simulink model "sensorModel"  (R2025b)
settings: Solver=ode2  StartTime=0.0  StopTime=1  FixedStep=1/100  RelTol=1e-3  EnableMultiTasking=on
PreLoadFcn:
  | stepsize_sens = evalin('base', get_param(bdroot, 'FixedStep'));
undefined symbols (not defined in the file or in its folder): defaultConsts, DiscIntNeverNeededParam, sensors, vehicle
libraries: simulink x2, aerolibatmos2 x1
settings Model: Creator=ac112430  LastModifiedBy=ac124458
settings SolverCC: AlgebraicLoopSolver=TrustRegion
settings DataIOCC: ReturnWorkspaceOutputs=off
settings OptimizationCC: LifeSpan=inf
settings DebuggingCC: UnconnectedInputMsg=warning  UnconnectedOutputMsg=warning  UnconnectedLineMsg=warning  SFExecutionAtInitializationDiag=none  ArithmeticOperatorsInVariantConditions=warning
settings HardwareCC: ProdBitPerSizeT=32.0  ProdBitPerPtrDiffT=32.0  ProdWordSize=32.0  ProdHWDeviceType=Specified
settings ModelReferenceCC: EnableRefExpFcnMdlSchedulingChecks=on  ModelReferenceNumInstancesAllowed=Single
settings SFSimCC: SimUseLocalCustomCode=off  CustomCodeUndefinedFunction=UseInterfaceOnly
settings RTWCC: RTWUseLocalCustomCode=off  GPUComputeCapability=3.5
settings CodeAppCC: StateflowObjectComments=on
settings GRTTargetCC: SubcomponentCodeInterfacePackaging=Nonreusable function

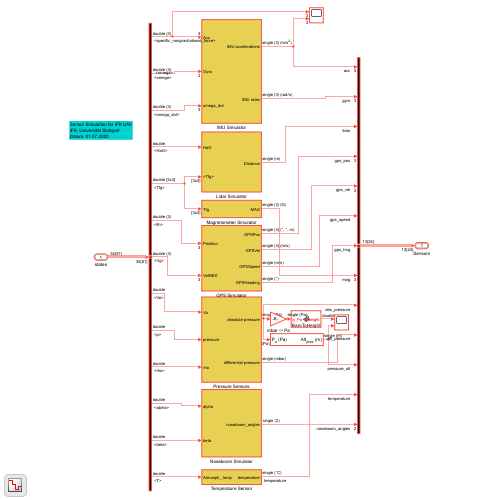
[thumbnail: Simulink's stored preview of the top-level diagram]
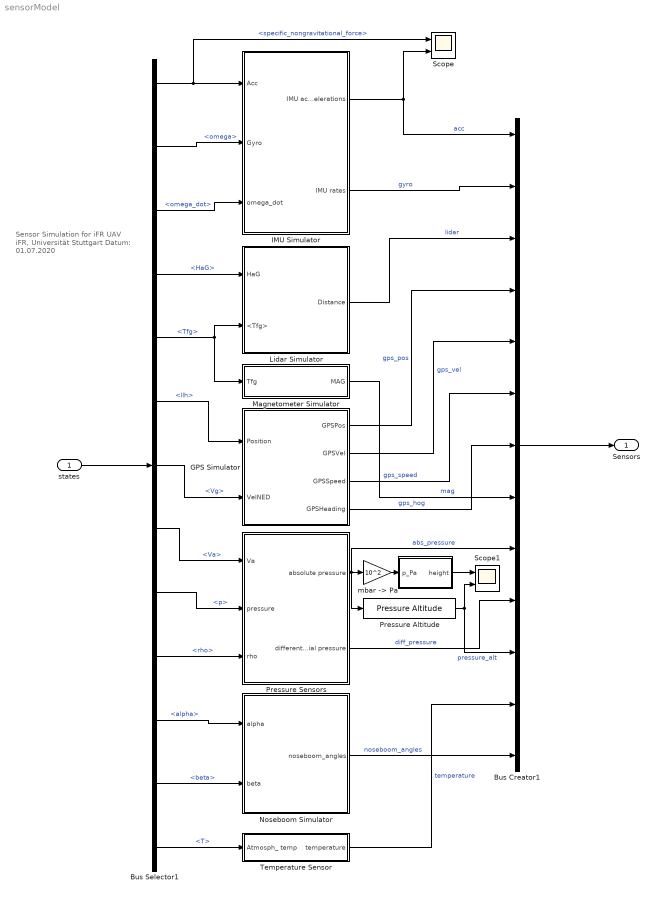
== system sensorModel ==
  note: Sensor Simulation for iFR UAV
      | iFR, Universität Stuttgart
      | Datum: 01.07.2020
  states : Inport  OutDataTypeStr=Bus: fmBus
  " " : MATLAB Function  TreatAsAtomicUnit=on
  Bus Creator1 : BusCreator  Inputs=13  OutDataTypeStr=Bus: sensorBus
      settings: InheritFromInputs=off
  Bus Selector1 : BusSelector  OutputSignals=utilityBus.specific_nongravitational_force,rigidbodyBus.omega,utilityBus.omega_dot,utilityBus.HaG,rigidbodyBus.Tfg,rigidbodyBus.llh,rigidbodyBus.Vg,atmosBus.Va,atmosBus.p,atmosBus.rho,atmosBus.alpha,atmosBus.beta,atmosBus.T
  GPS Simulator : Subsystem
  IMU Simulator : Subsystem
  Lidar Simulator : Subsystem
  Magnetometer Simulator : Subsystem
  Noseboom Simulator : Subsystem
  Pressure Altitude : aerolibatmos2/Pressure Altitude  units=Metric (MKS)  action=Warning
  Pressure Sensors : Subsystem
  Scope : Scope  NumInputPorts=2
      settings: ActiveDisplayYMinimum=-13.26607  ActiveDisplayYMaximum=18.32834
  Scope1 : Scope  NumInputPorts=2
      settings: DataLoggingVariableName=ScopeData2
  Temperature Sensor : Subsystem
  "mbar -> Pa" : Gain  Gain=10^2
  Sensors : Outport  OutDataTypeStr=Bus: sensorBus
  wires:
  Temperature Sensor/1(temperature) -> Bus Creator1/12  "temperature"
  Pressure Sensors/1(absolute pressure) -> Bus Creator1/9, Pressure Altitude/1, "mbar -> Pa"/1  "abs_pressure"
  GPS Simulator/2(GPSVel) -> Bus Creator1/5  "gps_vel"
  GPS Simulator/4(GPSHeading) -> Bus Creator1/7  "gps_hog"
  Magnetometer Simulator/1(MAG) -> Bus Creator1/8  "mag"
  Pressure Sensors/2(differential pressure) -> Bus Creator1/10  "diff_pressure"
  IMU Simulator/1(IMU accelerations) -> Bus Creator1/1, Scope/2  "acc"
  IMU Simulator/2(IMU rates) -> Bus Creator1/2  "gyro"
  Pressure Altitude/1 -> Bus Creator1/11, Scope1/2  "pressure_alt"
  Noseboom Simulator/1(noseboom_angles) -> Bus Creator1/13  "noseboom_angles"
  GPS Simulator/3(GPSSpeed) -> Bus Creator1/6  "gps_speed"
  GPS Simulator/1(GPSPos) -> Bus Creator1/4  "gps_pos"
  Bus Selector1/3 -> IMU Simulator/3(omega_dot)  "<omega_dot>"
  Bus Selector1/2 -> IMU Simulator/2(Gyro)  "<omega>"
  Bus Selector1/11 -> Noseboom Simulator/1(alpha)  "<alpha>"
  Bus Selector1/12 -> Noseboom Simulator/2(beta)  "<beta>"
  Bus Selector1/10 -> Pressure Sensors/3(rho)  "<rho>"
  states/1 -> Bus Selector1/1
  Bus Selector1/6 -> GPS Simulator/1(Position)  "<llh>"
  Bus Selector1/9 -> Pressure Sensors/2(pressure)  "<p>"
  Bus Selector1/5 -> Lidar Simulator/2(<Tfg>), Magnetometer Simulator/1(Tfg)  "<Tfg>"
  Bus Selector1/4 -> Lidar Simulator/1(HaG)  "<HaG>"
  Bus Selector1/8 -> Pressure Sensors/1(Va)  "<Va>"
  Bus Selector1/7 -> GPS Simulator/2(VelNED)  "<Vg>"
  Bus Selector1/1 -> Scope/1, IMU Simulator/1(Acc)  "<specific_nongravitational_force>"
  Bus Selector1/13 -> Temperature Sensor/1(Atmosph_ temp)  "<T>"
  Lidar Simulator/1(Distance) -> Bus Creator1/3  "lidar"
  "mbar -> Pa"/1 -> " "/1(p_Pa)
  " "/1(height) -> Scope1/1
  Bus Creator1/1 -> Sensors/1

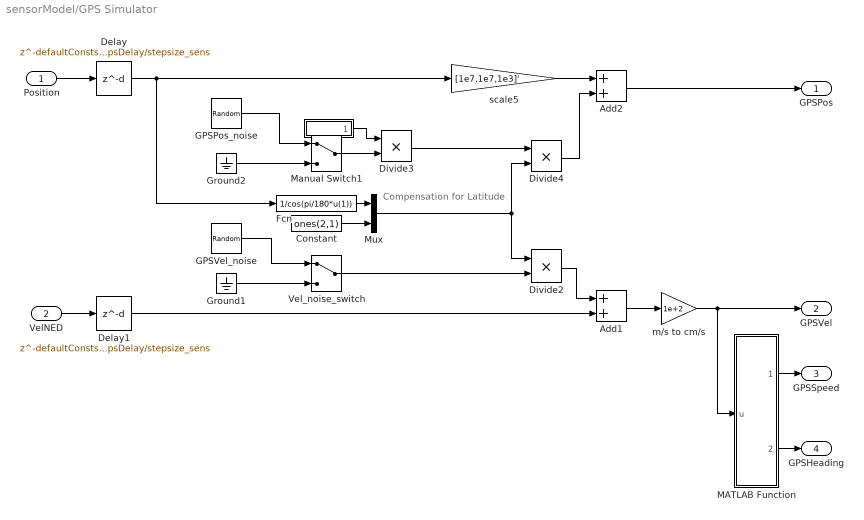
== system sensorModel/GPS Simulator ==
  note: Compensation for Latitude
  Position : Inport
  VelNED : Inport  Port=2
  "  " : MATLAB Function  TreatAsAtomicUnit=on
  Add1 : Sum
  Add2 : Sum  OutDataTypeStr=single
  Constant : Constant  Value=ones(2,1)
  Delay : Delay  DelayLength=defaultConsts.gpsDelay/stepsize_sens  InitialCondition=vehicle.pos0'*ones(1,defaultConsts.gpsDelay/stepsize_sens)
  Delay1 : Delay  DelayLength=defaultConsts.gpsDelay/stepsize_sens  InitialCondition=vehicle.pos0'*ones(1,defaultConsts.gpsDelay/stepsize_sens)
  Divide2 : Product  Inputs=**
  Divide3 : Product  Inputs=**
  Divide4 : Product  Inputs=**
  Fcn : Fcn  Expr=1/cos(pi/180*u(1))
  GPSPos_noise : RandomNumber  Variance=sensors.gps.sigmaPos.^2  Seed=[24522 237487 32748]
  GPSVel_noise : RandomNumber  Variance=sensors.gps.sigmaVel.^2  Seed=[127 2778 1883]
  Ground1 : Ground
  Ground2 : Ground
  MATLAB Function : MATLAB Function  TreatAsAtomicUnit=on
  Manual Switch1 : ManualSwitch
  Mux : Mux  Inputs=2
  Vel_noise_switch : ManualSwitch
  m/s to cm/s : Gain  Gain=1e+2  OutDataTypeStr=single
  scale5 : Gain  Gain=[1e7,1e7,1e3]'
  GPSPos : Outport  OutDataTypeStr=single  VectorParamsAs1DForOutWhenUnconnected=off
  GPSVel : Outport  Port=2  OutDataTypeStr=single  VectorParamsAs1DForOutWhenUnconnected=off
  GPSSpeed : Outport  Port=3  OutDataTypeStr=single  VectorParamsAs1DForOutWhenUnconnected=off
  GPSHeading : Outport  Port=4  OutDataTypeStr=single  VectorParamsAs1DForOutWhenUnconnected=off
  wires:
  Vel_noise_switch/1 -> Divide2/2
  Add1/1 -> m/s to cm/s/1
  VelNED/1 -> Delay1/1
  GPSVel_noise/1 -> Vel_noise_switch/1
  Ground1/1 -> Vel_noise_switch/2
  Delay1/1 -> Add1/2
  Manual Switch1/1 -> Divide3/2
  Delay/1 -> scale5/1, Fcn/1
  Position/1 -> Delay/1
  Ground2/1 -> Manual Switch1/2
  Mux/1 -> Divide2/1, Divide4/2
  Add2/1 -> GPSPos/1
  m/s to cm/s/1 -> GPSVel/1, MATLAB Function/1(u)
  MATLAB Function/1(speed) -> GPSSpeed/1
  MATLAB Function/2(heading) -> GPSHeading/1
  Divide2/1 -> Add1/1
  Divide3/1 -> Divide4/1
  GPSPos_noise/1 -> Manual Switch1/1
  Divide4/1 -> Add2/2
  Fcn/1 -> Mux/1
  Constant/1 -> Mux/2
  scale5/1 -> Add2/1
  "  "/1(ned2lla) -> Divide3/1

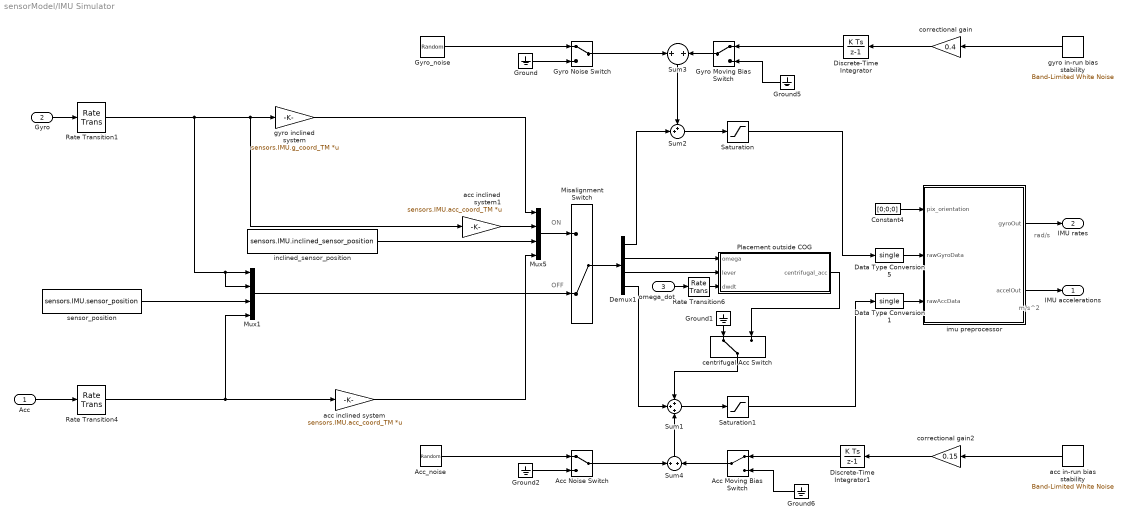
== system sensorModel/IMU Simulator ==
  note: ON
  note: OFF
  note: rad/s
  note: m/s^2
  Acc : Inport
  Gyro : Inport  Port=2
  omega_dot : Inport  Port=3
  Acc Moving Bias Switch : ManualSwitch
  Acc Noise Switch : ManualSwitch
  Acc_noise : RandomNumber  Mean=sensors.IMU.acc_initial_bias  Variance=sensors.IMU.acc_noise^2*[1 1 1]  Seed=[6 7 8]  SampleTime=sensors.IMU.timestep
  Constant4 : Constant  Value=[0;0;0]  OutDataTypeStr=single
  Data Type Conversion1 : DataTypeConversion  OutDataTypeStr=single  SaturateOnIntegerOverflow=off  RndMeth=Floor
  Data Type Conversion5 : DataTypeConversion  OutDataTypeStr=single  SaturateOnIntegerOverflow=off  RndMeth=Floor
  Demux1 : Demux
  Discrete-Time Integrator : DiscreteIntegrator  SampleTime=-1  ICPrevOutput=DiscIntNeverNeededParam  ICPrevScaledInput=DiscIntNeverNeededParam
  Discrete-Time Integrator1 : DiscreteIntegrator  SampleTime=-1  ICPrevOutput=DiscIntNeverNeededParam  ICPrevScaledInput=DiscIntNeverNeededParam
  Ground{,1..2,5..6} (5 alike) : Ground
  Gyro Moving Bias Switch : ManualSwitch
  Gyro Noise Switch : ManualSwitch
  Gyro_noise : RandomNumber  Mean=sensors.IMU.g_initial_bias  Variance=sensors.IMU.g_noise^2*[1 1 1]  Seed=[0 1 2]  SampleTime=sensors.IMU.timestep
  Misalignment Switch : ManualSwitch  CurrentSetting=0
  Mux1 : Mux
  Mux5 : Mux
  Placement outside COG : MATLAB Function  TreatAsAtomicUnit=on
  Rate Transition1 : RateTransition  OutPortSampleTime=sensors.IMU.timestep
  Rate Transition4 : RateTransition  OutPortSampleTime=sensors.IMU.timestep
  Rate Transition6 : RateTransition  OutPortSampleTime=stepsize_sens
  Saturation : Saturate  UpperLimit=sensors.IMU.g_range  LowerLimit=-sensors.IMU.g_range
  Saturation1 : Saturate  UpperLimit=sensors.IMU.acc_range  LowerLimit=-sensors.IMU.acc_range
  Sum1 : Sum  Inputs=+++
  Sum2 : Sum  Inputs=++|
  Sum3 : Sum
  Sum4 : Sum
  acc in-run bias stability : simulink/Sources/Band-Limited White Noise  Cov=sensors.IMU.acc_inrun_bias^2*[1 1 1]  Ts=sensors.IMU.timestep  seed=[40 31 56]
  acc inclined system : Gain  Gain=sensors.IMU.acc_coord_TM  Multiplication=Matrix(K*u)
  acc inclined system1 : Gain  Gain=sensors.IMU.acc_coord_TM  Multiplication=Matrix(K*u)
  centrifugal Acc Switch : ManualSwitch
  correctional gain : Gain  Gain=0.4
  correctional gain2 : Gain  Gain=0.15
  gyro in-run bias stability : simulink/Sources/Band-Limited White Noise  Cov=sensors.IMU.g_inrun_bias^2*[1 1 1]  Ts=sensors.IMU.timestep  seed=[21 30 27]
  gyro inclined system : Gain  Gain=sensors.IMU.g_coord_TM  Multiplication=Matrix(K*u)
  imu preprocessor : MATLAB Function  TreatAsAtomicUnit=on
  inclined_sensor_position : Constant  Value=sensors.IMU.inclined_sensor_position
  sensor_position : Constant  Value=sensors.IMU.sensor_position
  IMU accelerations : Outport  VectorParamsAs1DForOutWhenUnconnected=off
  IMU rates : Outport  Port=2  VectorParamsAs1DForOutWhenUnconnected=off
  wires:
  Sum2/1 -> Saturation/1
  Sum1/1 -> Saturation1/1
  Ground/1 -> Gyro Noise Switch/2
  Ground2/1 -> Acc Noise Switch/2
  Acc/1 -> Rate Transition4/1
  Rate Transition4/1 -> Mux1/4, acc inclined system/1
  centrifugal Acc Switch/1 -> Sum1/1
  Gyro/1 -> Rate Transition1/1
  Demux1/1 -> Sum2/2
  Ground1/1 -> centrifugal Acc Switch/1
  acc inclined system1/1 -> Mux5/2
  Misalignment Switch/1 -> Demux1/1
  acc inclined system/1 -> Mux5/4
  Mux1/1 -> Misalignment Switch/2
  Mux5/1 -> Misalignment Switch/1
  gyro inclined system/1 -> Mux5/1
  Demux1/4 -> Sum1/2
  Demux1/3 -> Placement outside COG/2(lever)
  inclined_sensor_position/1 -> Mux5/3
  Rate Transition1/1 -> gyro inclined system/1, acc inclined system1/1, Mux1/1, Mux1/2
  Gyro Noise Switch/1 -> Sum3/1
  Sum3/1 -> Sum2/1
  Acc Noise Switch/1 -> Sum4/1
  Sum4/1 -> Sum1/3
  Saturation/1 -> Data Type Conversion5/1
  Ground6/1 -> Acc Moving Bias Switch/2
  Discrete-Time Integrator1/1 -> Acc Moving Bias Switch/1
  Discrete-Time Integrator/1 -> Gyro Moving Bias Switch/1
  Ground5/1 -> Gyro Moving Bias Switch/2
  correctional gain/1 -> Discrete-Time Integrator/1
  Acc_noise/1 -> Acc Noise Switch/1
  Gyro_noise/1 -> Gyro Noise Switch/1
  gyro in-run bias stability/1 -> correctional gain/1
  acc in-run bias stability/1 -> correctional gain2/1
  Saturation1/1 -> Data Type Conversion1/1
  sensor_position/1 -> Mux1/3
  Demux1/2 -> Placement outside COG/1(omega)
  Placement outside COG/1(centrifugal_acc) -> centrifugal Acc Switch/2
  correctional gain2/1 -> Discrete-Time Integrator1/1
  Gyro Moving Bias Switch/1 -> Sum3/2
  Acc Moving Bias Switch/1 -> Sum4/2
  omega_dot/1 -> Rate Transition6/1
  Rate Transition6/1 -> Placement outside COG/3(dwdt)
  Data Type Conversion5/1 -> imu preprocessor/2(rawGyroData)
  Data Type Conversion1/1 -> imu preprocessor/3(rawAccData)
  Constant4/1 -> imu preprocessor/1(pix_orientation)
  imu preprocessor/1(gyroOut) -> IMU rates/1
  imu preprocessor/2(accelOut) -> IMU accelerations/1

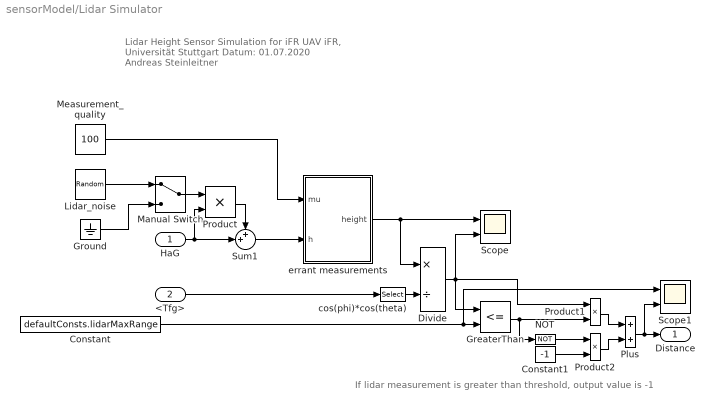
== system sensorModel/Lidar Simulator ==
  note: If lidar measurement is greater than threshold, output value is -1
  note: Lidar Height Sensor Simulation for iFR UAV
      | iFR, Universität Stuttgart
      | Datum: 01.07.2020
      |
      | Andreas Steinleitner
  HaG : Inport
  <Tfg> : Inport  Port=2
  Constant : Constant  Value=defaultConsts.lidarMaxRange
  Constant1 : Constant  Value=-1
  Divide : Product  Inputs=*/
  GreaterThan : RelationalOperator  Operator=<=  OutDataTypeStr=boolean  RndMeth=Simplest  InputSameDT=off
  Ground : Ground
  Lidar_noise : RandomNumber  Variance=sensors.lidar.sigma^2  Seed=29741  SampleTime=stepsize_sens
  Manual Switch : ManualSwitch
  Measurement_quality : Constant  Value=100
  NOT : Logic  Operator=NOT  AllPortsSameDT=off  OutDataTypeStr=boolean
  Plus : Sum  OutDataTypeStr=single
  Product : Product
  Product1 : Product
  Product2 : Product
  Scope : Scope  NumInputPorts=2
      settings: ActiveDisplayYMinimum=-38.99101  ActiveDisplayYMaximum=350.9191
  Scope1 : Scope  NumInputPorts=2
      settings: DataLoggingVariableName=ScopeData3
  Sum1 : Sum  Inputs=++|
  cos(phi)*cos(theta) : Selector  NumberOfDimensions=2  InputPortWidth=3  IndexOptions=Index vector (dialog),Index vector (dialog)  Indices=3,3  OutputSizes=1,1
  errant measurements : MATLAB Function  TreatAsAtomicUnit=on
  Distance : Outport  VectorParamsAs1DForOutWhenUnconnected=off
  wires:
  HaG/1 -> Product/2, Sum1/2
  Ground/1 -> Manual Switch/2
  Lidar_noise/1 -> Manual Switch/1
  Manual Switch/1 -> Product/1
  Product/1 -> Sum1/1
  <Tfg>/1 -> cos(phi)*cos(theta)/1
  cos(phi)*cos(theta)/1 -> Divide/2
  Measurement_quality/1 -> errant measurements/1(mu)
  Sum1/1 -> errant measurements/2(h)
  errant measurements/1(height) -> Scope/1, Divide/1
  Divide/1 -> Scope/2, GreaterThan/1, Product1/1
  Constant/1 -> Scope1/1, GreaterThan/2
  GreaterThan/1 -> NOT/1, Product1/2
  NOT/1 -> Product2/1
  Constant1/1 -> Product2/2
  Product1/1 -> Plus/1
  Product2/1 -> Plus/2
  Plus/1 -> Scope1/2, Distance/1

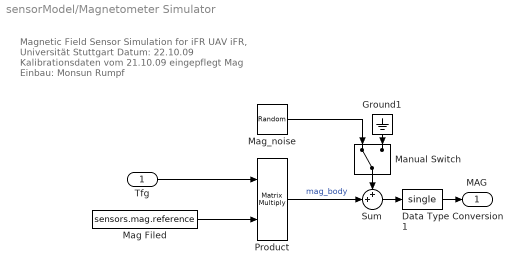
== system sensorModel/Magnetometer Simulator ==
  note: Magnetic Field Sensor Simulation for iFR UAV
      | iFR, Universität Stuttgart
      | Datum: 22.10.09
      |
      | Kalibrationsdaten vom 21.10.09 eingepflegt
      | Mag Einbau: Monsun Rumpf
  Tfg : Inport
  Data Type Conversion1 : DataTypeConversion  OutDataTypeStr=single  SaturateOnIntegerOverflow=off  RndMeth=Floor
  Ground1 : Ground
  Mag Filed : Constant  Value=sensors.mag.reference
  Mag_noise : RandomNumber  Variance=sensors.mag.sigma^2  Seed=[78234 3274 28736]  SampleTime=stepsize_sens
  Manual Switch : ManualSwitch
  Product : Product  Multiplication=Matrix(*)
  Sum : Sum  Inputs=++|
  MAG : Outport  VectorParamsAs1DForOutWhenUnconnected=off
  wires:
  Tfg/1 -> Product/1
  Product/1 -> Sum/2  "mag_body"
  Mag Filed/1 -> Product/2
  Sum/1 -> Data Type Conversion1/1
  Ground1/1 -> Manual Switch/2
  Mag_noise/1 -> Manual Switch/1
  Manual Switch/1 -> Sum/1
  Data Type Conversion1/1 -> MAG/1

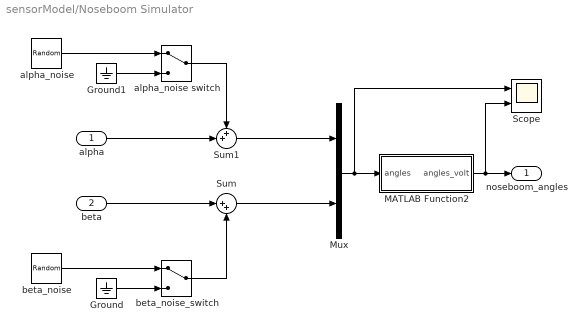
== system sensorModel/Noseboom Simulator ==
  alpha : Inport
  beta : Inport  Port=2
  Ground : Ground
  Ground1 : Ground
  MATLAB Function2 : MATLAB Function  TreatAsAtomicUnit=on
  Mux : Mux  Inputs=2
  Scope : Scope  NumInputPorts=2
      settings: ActiveDisplayYMinimum=-1.15354  ActiveDisplayYMaximum=0.87545
  Sum : Sum  Inputs=|++
  Sum1 : Sum  Inputs=++|
  alpha_noise : RandomNumber  Variance=deg2rad(0.5)^2  SampleTime=stepsize_sens
  alpha_noise switch : ManualSwitch
  beta_noise : RandomNumber  Variance=deg2rad(0.5)^2  SampleTime=stepsize_sens
  beta_noise_switch : ManualSwitch
  noseboom_angles : Outport  VectorParamsAs1DForOutWhenUnconnected=off
  wires:
  alpha/1 -> Sum1/2
  Sum1/1 -> Mux/1
  beta/1 -> Sum/1
  alpha_noise switch/1 -> Sum1/1
  beta_noise_switch/1 -> Sum/2
  Sum/1 -> Mux/2
  alpha_noise/1 -> alpha_noise switch/1
  beta_noise/1 -> beta_noise_switch/1
  Ground1/1 -> alpha_noise switch/2
  Ground/1 -> beta_noise_switch/2
  Mux/1 -> Scope/1, MATLAB Function2/1(angles)
  MATLAB Function2/1(angles_volt) -> Scope/2, noseboom_angles/1

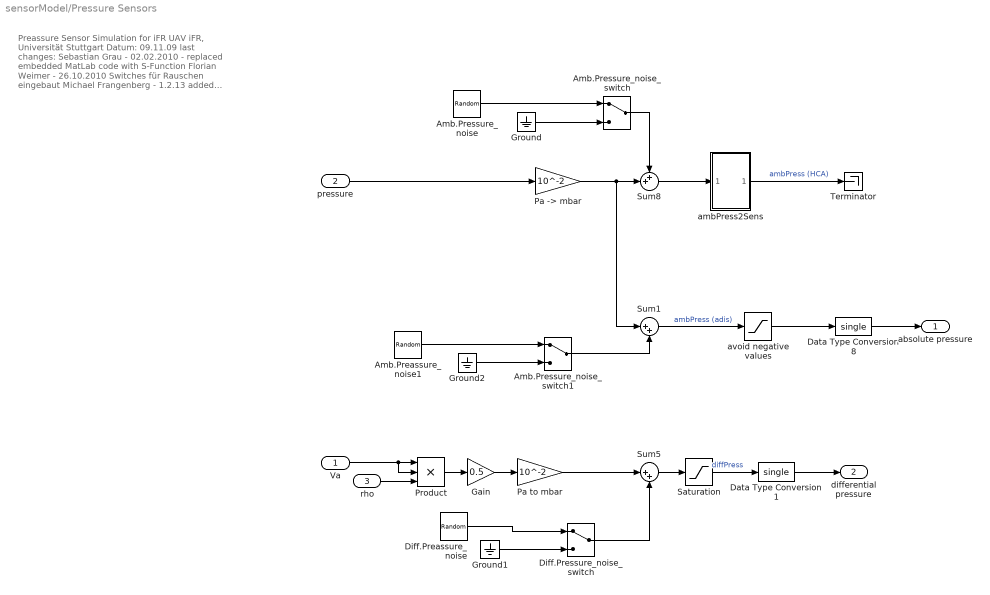
== system sensorModel/Pressure Sensors ==
  note: Preassure Sensor Simulation for iFR UAV
      | iFR, Universität Stuttgart
      | Datum: 09.11.09
      |
      | last changes:
      | Sebastian Grau - 02.02.2010 - replaced
      | embedded MatLab code with S-Function
      | Florian Weimer - 26.10.2010 Switches für
      | Rauschen eingebaut
      | Michael Frangenberg - 1.2.13 added ADIS baro
      |
      | Comments:
      | - add random walk process to sensors
  Va : Inport
  pressure : Inport  Port=2
  rho : Inport  Port=3
  Amb.Preassure_noise1 : RandomNumber  Variance=sensors.airData.sigmaAdis^2  Seed=6234  SampleTime=stepsize_sens
  Amb.Pressure_noise : RandomNumber  Variance=sensors.airData.sigmaHCA^2  Seed=29741  SampleTime=stepsize_sens
  Amb.Pressure_noise_switch : ManualSwitch
  Amb.Pressure_noise_switch1 : ManualSwitch
  Data Type Conversion1 : DataTypeConversion  OutDataTypeStr=single  SaturateOnIntegerOverflow=off  RndMeth=Floor
  Data Type Conversion8 : DataTypeConversion  OutDataTypeStr=single  SaturateOnIntegerOverflow=off  RndMeth=Floor
  Diff.Preassure_noise : RandomNumber  Variance=sensors.airData.sigmaDiff^2  Seed=237  SampleTime=stepsize_sens
  Diff.Pressure_noise_switch : ManualSwitch
  Gain : Gain  Gain=0.5
  Ground : Ground
  Ground1 : Ground
  Ground2 : Ground
  "Pa -> mbar" : Gain  Gain=10^-2
  Pa to mbar : Gain  Gain=10^-2
  Product : Product  Inputs=3
  Saturation : Saturate  UpperLimit=inf  LowerLimit=0.05
  Sum1 : Sum  Inputs=|++
  Sum5 : Sum  Inputs=|++
  Sum8 : Sum  Inputs=++|
  Terminator : Terminator
  ambPress2Sens : Subsystem
  avoid negative values : Saturate  UpperLimit=100000000000  LowerLimit=0.1
  absolute pressure : Outport  VectorParamsAs1DForOutWhenUnconnected=off
  differential pressure : Outport  Port=2  VectorParamsAs1DForOutWhenUnconnected=off
  wires:
  Diff.Pressure_noise_switch/1 -> Sum5/2
  Amb.Pressure_noise_switch/1 -> Sum8/1
  Sum8/1 -> ambPress2Sens/1(In1)
  Sum5/1 -> Saturation/1
  ambPress2Sens/1(Out1) -> Terminator/1  "ambPress (HCA)"
  Saturation/1 -> Data Type Conversion1/1  "diffPress"
  Amb.Pressure_noise/1 -> Amb.Pressure_noise_switch/1
  Ground/1 -> Amb.Pressure_noise_switch/2
  Diff.Preassure_noise/1 -> Diff.Pressure_noise_switch/1
  Ground1/1 -> Diff.Pressure_noise_switch/2
  Amb.Pressure_noise_switch1/1 -> Sum1/2
  Amb.Preassure_noise1/1 -> Amb.Pressure_noise_switch1/1
  Ground2/1 -> Amb.Pressure_noise_switch1/2
  Sum1/1 -> avoid negative values/1  "ambPress (adis)"
  pressure/1 -> "Pa -> mbar"/1
  Va/1 -> Product/2, Product/1
  rho/1 -> Product/3
  Product/1 -> Gain/1
  Gain/1 -> Pa to mbar/1
  Pa to mbar/1 -> Sum5/1
  "Pa -> mbar"/1 -> Sum1/1, Sum8/2
  Data Type Conversion8/1 -> absolute pressure/1
  Data Type Conversion1/1 -> differential pressure/1
  avoid negative values/1 -> Data Type Conversion8/1

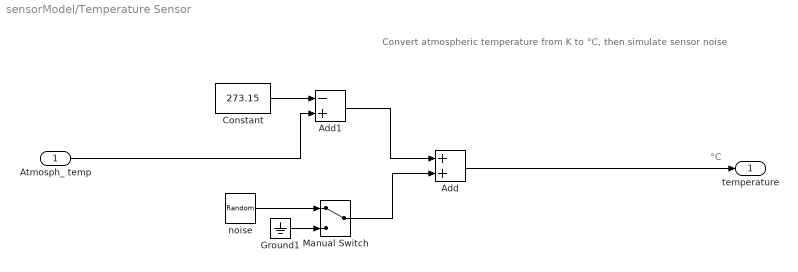
== system sensorModel/Temperature Sensor ==
  note: °C
  note: Convert atmospheric temperature from K to °C, then simulate sensor noise
  Atmosph_ temp : Inport
  Add : Sum  OutDataTypeStr=single
  Add1 : Sum  Inputs=-+  OutDataTypeStr=double
  Constant : Constant  Value=273.15
  Ground1 : Ground
  Manual Switch : ManualSwitch
  noise : RandomNumber  Variance=0.1^2  SampleTime=0.01
  temperature : Outport  OutDataTypeStr=single  VectorParamsAs1DForOutWhenUnconnected=off
  wires:
  Add/1 -> temperature/1
  Constant/1 -> Add1/1
  Atmosph_ temp/1 -> Add1/2
  Add1/1 -> Add/1
  Manual Switch/1 -> Add/2
  Ground1/1 -> Manual Switch/2
  noise/1 -> Manual Switch/1

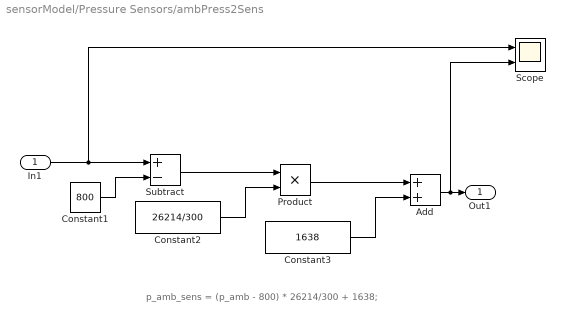
== system sensorModel/Pressure Sensors/ambPress2Sens ==
  note: p_amb_sens = (p_amb - 800) * 26214/300 + 1638;
  In1 : Inport
  Add : Sum
  Constant1 : Constant  Value=800
  Constant2 : Constant  Value=26214/300
  Constant3 : Constant  Value=1638
  Product : Product  RndMeth=Zero
  Scope : Scope  NumInputPorts=2
      settings: ActiveDisplayYMinimum=944.51744  ActiveDisplayYMaximum=961.03031
  Subtract : Sum  Inputs=+-
  Out1 : Outport  VectorParamsAs1DForOutWhenUnconnected=off
  wires:
  Subtract/1 -> Product/1
  Product/1 -> Add/1
  Constant3/1 -> Add/2
  Constant2/1 -> Product/2
  Constant1/1 -> Subtract/2
  In1/1 -> Scope/1, Subtract/1
  Add/1 -> Scope/2, Out1/1

== matlab function sensorModel/IMU Simulator/Placement outside COG ==
  data: omega input; centrifugal_acc output; lever input; dwdt input
function centrifugal_acc = fcn(omega, lever, dwdt)

%centrifugal acceleration is -omega x(omega x lever)
centrifugal_acc = zeros(3,1);
centrifugal_acc = cross(omega,cross(omega,lever)) + cross(dwdt, lever);

== matlab function sensorModel/GPS Simulator/MATLAB Function ==
  data: u input; speed output single; heading output single
function [speed,heading] = fcn(u)

speed = norm(u);
heading = atan2(u(2),u(1));

== matlab function sensorModel/Lidar Simulator/errant measurements ==
  data: mu input; h input; height output; sensors parameter
function height = fcn(mu,h,sensors)

maxHeight = 50;
height = h;

errorFreq = min(h,maxHeight)/(mu*100);
if rand()<errorFreq
    height = round(rand()*10)*h;
end

if h > maxHeight
    height = rand_generator(sensors.lidar.pdf.x,sensors.lidar.pdf.Fx);
end
end

function rand_num = rand_generator(grid,val)
splitter = rand(1,1);
rand_var = rand(1,1);
segment_idx = find(splitter<val,1);
rand_num = rand_var*(grid(segment_idx)-grid(segment_idx-1))+grid(segment_idx-1);
rand_num = rand_num(1,1);
end

== matlab function sensorModel/GPS Simulator/   ==
  settings: updateMethod=DISCRETE
  data: ned2lla output; defaultConsts parameter size=1
function ned2lla = converter(defaultConsts)
semiMajorAxis = single(6378137);
eccentricity = single(8.1819190842622e-2);
R0 = semiMajorAxis/sqrt(1-eccentricity^2*sin(defaultConsts.initialPositionLla(1)*pi/180)^2);
ned2lla = 1./([(1-eccentricity^2)/semiMajorAxis^2*R0^3+defaultConsts.initialPositionLla(3); (R0+defaultConsts.initialPositionLla(3))*cos(defaultConsts.initialPositionLla(1)*pi/180); -1].*single([1e-7*pi/180; 1e-7*pi/180; 1e-3]));
% refLlhPosRaw=int32([defaultConsts.initialPositionLla(1:2)*1e7; defaultConsts.initialPositionLla(3)*1e3]);
%     semiMajorAxis=single(6378137);
%     eccentricity=single(8.1819190842622e-2);
%     posScaleFactor=single([1e-7*pi/180; 1e-7*pi/180; 1e-3]);
%     lattitudeRef=posScaleFactor(1)*single(refLlhPosRaw(1));
%     heightRef=posScaleFactor(3)*single(refLlhPosRaw(3));
%     R0=semiMajorAxis/sqrt(1-eccentricity^2*sin(lattitudeRef)^2);
%     ned2lla=1./[(1-eccentricity^2)/semiMajorAxis^2*R0^3+heightRef; (R0+heightRef)*cos(lattitudeRef); -1].*posScaleFactor;
end

== matlab function sensorModel/  ==
  data: p_Pa input; height output; defaultConsts parameter
function height=BaroToHeight(p_Pa, defaultConsts)
    
    height_uncorrected = computeHeightFromPressure(p_Pa, defaultConsts);
    
    height = height_uncorrected;%-defaultConsts.initialPositionLla(3);
end

function height_calc = computeHeightFromPressure(pressure, constants)
    height_calc = double(constants.referenceTemperature/constants.temperatureGradient*(1-(pressure/constants.referencePressure)^((constants.atmosphereKappa-1)/constants.atmosphereKappa)));
end

== matlab function sensorModel/Noseboom Simulator/MATLAB Function2 ==
  data: angles input; angles_volt output single
function angles_volt  = rad2volt(angles)

alpha_v = (angles(1)+3.5651)/1.9428;
beta_v = (angles(2)+2.8122)/2.3954;

angles_volt=single([alpha_v;beta_v]);

== matlab function sensorModel/IMU Simulator/imu preprocessor ==
  settings: updateMethod=DISCRETE
  data: pix_orientation input single; gyroOut output single size=3; rawGyroData input single; accelOut output single size=3; rawAccData input single size=3
function [gyroOut,accelOut]=preprocessImuData(pix_orientation,rawGyroData,rawAccData)

T1 = [1 0 0;0 cos(pix_orientation(1)) sin(pix_orientation(1));0 -sin(pix_orientation(1)) cos(pix_orientation(1))];
T2 = [cos(pix_orientation(2)) 0 -sin(pix_orientation(2));0 1 0;sin(pix_orientation(2)) 0 cos(pix_orientation(2))];
T3 = [cos(pix_orientation(3)) sin(pix_orientation(3)) 0;-sin(pix_orientation(3)) cos(pix_orientation(3)) 0;0 0 1];
T = T3'*T2'*T1';

gyroOut= T*rawGyroData;
accelOut= T*rawAccData;
